simulink model "SMA_displacementIn_PC2"  (R2018a)
settings: Solver=ode15s  StartTime=0.0  StopTime=100  RelTol=1e-8  AbsTol=1e-8  EnableMultiTasking=on
libraries: simulink x1
settings Model: Creator=Gianluca  LastModifiedBy=Matthias
settings SolverCC: AutoScaleAbsTol=off
settings DataIOCC: LimitDataPoints=on  SaveFormat=Array
settings OptimizationCC: LifeSpan=inf
settings DebuggingCC: UnderspecifiedInitializationDetection=Classic  MergeDetectMultiDrivingBlocksExec=none  SolverPrmCheckMsg=warning  StateNameClashWarn=warning  SFUnexpectedBacktrackingDiag=warning  SFNoUnconditionalDefaultTransitionDiag=warning  SFExecutionAtInitializationDiag=none
settings HardwareCC: ProdBitPerPointer=32  ProdBitPerSizeT=32  ProdBitPerPtrDiffT=32  ProdLargestAtomicFloat=None  ProdIntDivRoundTo=Undefined  ProdEndianess=Unspecified  ProdWordSize=32  ProdHWDeviceType=32-bit Generic
settings ModelReferenceCC: PropagateSignalLabelsOutOfModel=off
settings CodeAppCC: StateflowObjectComments=on
settings GRTTargetCC: TargetLangStandard=C89/C90 (ANSI)  GeneratePreprocessorConditionals=Disable all
settings ConfigComp: CovMetricSettings=dw  CovHtmlReporting=on  CovSaveCumulativeToWorkspaceVar=on  CovSaveSingleToWorkspaceVar=on  CovExternalEMLEnable=off

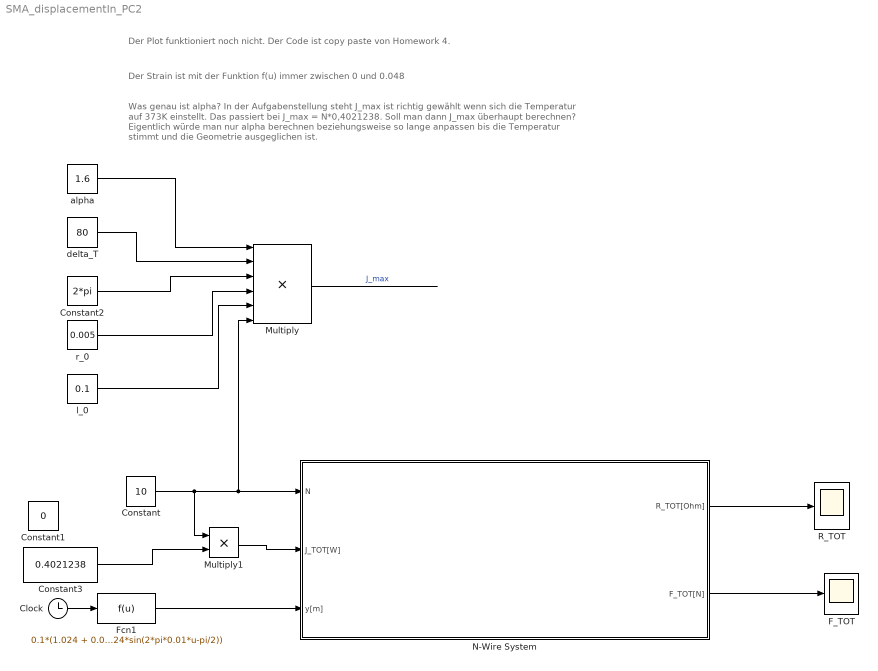
== system SMA_displacementIn_PC2 ==
  note: Der Plot funktioniert noch nicht. Der Code ist copy paste von Homework 4.
  note: Der Strain ist mit der Funktion f(u) immer zwischen 0 und 0.048
  note: Was genau ist alpha?
      | In der Aufgabenstellung steht J_max ist richtig gewählt wenn sich die Temperatur auf 373K einstellt.
      | Das passiert bei J_max = N*0,4021238. Soll man dann J_max überhaupt berechnen?
      | Eigentlich würde man nur alpha berechnen beziehungsweise so lange anpassen bis die Temperatur stimmt und die Geometrie ausgeglichen ist.
  Clock : Clock
  Constant : Constant  Value=10
  Constant1 : Constant  Value=0
  Constant2 : Constant  Value=2*pi
  Constant3 : Constant  Value=0.4021238
  "F_TOT " : Scope
  Fcn1 : Fcn  Expr=0.1*(1.024 + 0.024*sin(2*pi*0.01*u-pi/2))
  Multiply : Product  Inputs=6
  Multiply1 : Product
  "N-Wire System " : Subsystem
  R_TOT : Scope
  alpha : Constant  Value=1.6
  delta_T : Constant  Value=80
  l_0 : Constant  Value=0.1
  r_0 : Constant  Value=0.005
  wires:
  Constant/1 -> Multiply1/1, Multiply/6, "N-Wire System "/1(N)
  Clock/1 -> Fcn1/1
  Fcn1/1 -> "N-Wire System "/3(y[m])
  "N-Wire System "/1(R_TOT[Ohm]) -> R_TOT/1
  "N-Wire System "/2("F_TOT[N] ") -> "F_TOT "/1
  alpha/1 -> Multiply/1
  delta_T/1 -> Multiply/2
  Constant2/1 -> Multiply/3
  r_0/1 -> Multiply/4
  l_0/1 -> Multiply/5
  Multiply/1 -> ?  "J_max"
  Multiply1/1 -> "N-Wire System "/2("J_TOT[W] ")
  Constant3/1 -> Multiply1/2

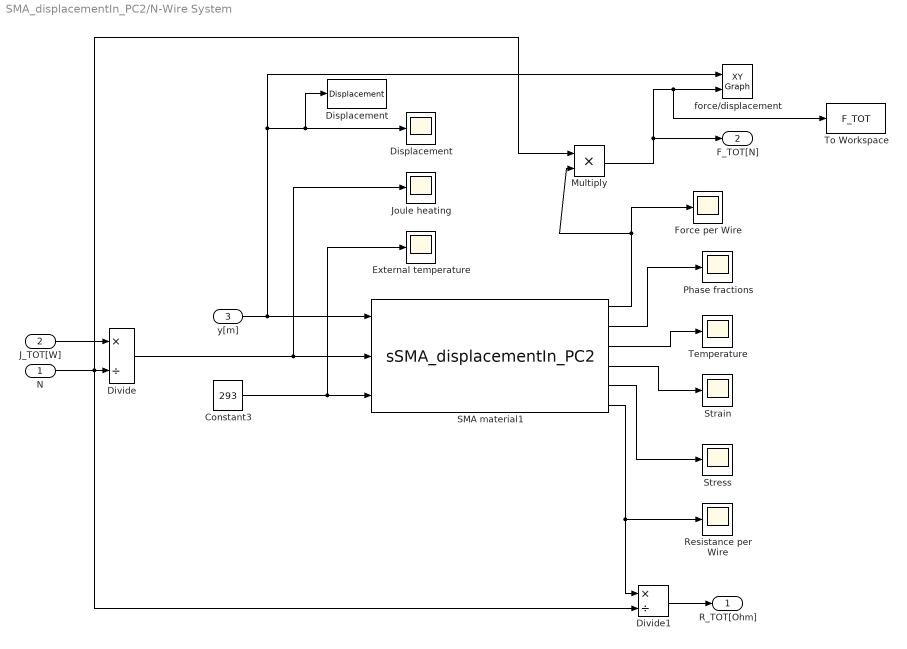
== system SMA_displacementIn_PC2/N-Wire System  ==
  N : Inport
  "J_TOT[W] " : Inport  Port=2
  y[m] : Inport  Port=3
  Constant3 : Constant  Value=293
  Displacement : Scope
  "Displacement " : ToWorkspace  VariableName=Displacement  SampleTime=-1
  Divide : Product  Inputs=*/
  Divide1 : Product  Inputs=*/
  External temperature : Scope
  "Force per Wire " : Scope
  Joule heating : Scope
  Multiply : Product
  Phase fractions : Scope
  Resistance per Wire : Scope
  SMA material1 : M-S-Function  FunctionName=sSMA_displacementIn_PC2  Parameters=params_PC2, initConds_PC2
      mask Display:
      | color('black');
      | patch(3*[-1 1 1 -1],1.1*[-1 -1 1 1],[1 1 1]);
      | patch([-1.6 -0.8],[-0.9 0.3],[0 0 0]);
      | patch([-0.8 1.2],[0.3 0.3],[0 0 0]);
      | patch([1.6 0.8],[0.9 -0.3],[0 0 0]);
      | patch([0.8 -1.2],[-0.3 -0.3],[0 0 0]);
      | disp('SMA');
      | 
      | color('blue');
      | port_label('input', 1, 'y [m]','texmode','on');
      | port_label('input', 2, 'J [W]','texmode','on');
      | port_label('input', 3, 'T_E [K]','texmode','on');
      | 
      | color('red');
      | port_label('output', 1, 'F [N]','texmode','on');
      | port_label('output', 2, 'x_+, x_-, x_A [-]','texmode','on');
      | port_label('output', 3, 'T [K]','texmode','on');
      | port_label('output', 4, '\epsilon [-]','texmode','on');
      | port_label('output', 5, '\sigma [Pa]','texmode','on');
      | port_label('output', 6, 'R [\Omega]','texmode','on');
  Strain : Scope
  Stress : Scope
  Temperature : Scope
  To Workspace : ToWorkspace  VariableName=F_TOT  SampleTime=-1
  force/displacement : simulink/Sinks/XY Graph  xmin=0.1  xmax=0.106  ymin=0  ymax=20  st=-1
  R_TOT[Ohm] : Outport
  "F_TOT[N] " : Outport  Port=2
  wires:
  SMA material1/6 -> Divide1/1, Resistance per Wire/1
  Constant3/1 -> SMA material1/3, External temperature/1
  Divide/1 -> Joule heating/1, SMA material1/2
  y[m]/1 -> SMA material1/1, force/displacement/1, "Displacement "/1, Displacement/1
  SMA material1/2 -> Phase fractions/1
  SMA material1/4 -> Strain/1
  SMA material1/1 -> Multiply/2, "Force per Wire "/1
  SMA material1/5 -> Stress/1
  SMA material1/3 -> Temperature/1
  "J_TOT[W] "/1 -> Divide/1
  N/1 -> Multiply/1, Divide/2, Divide1/2
  Multiply/1 -> "F_TOT[N] "/1, To Workspace/1, force/displacement/2
  Divide1/1 -> R_TOT[Ohm]/1
